simulink model "chap8_6sim"  (R2015a)
settings: Solver=ode45  StartTime=0.0  StopTime=30  RelTol=1e-3
settings Model: Creator=zhr  LastModifiedBy=zhr

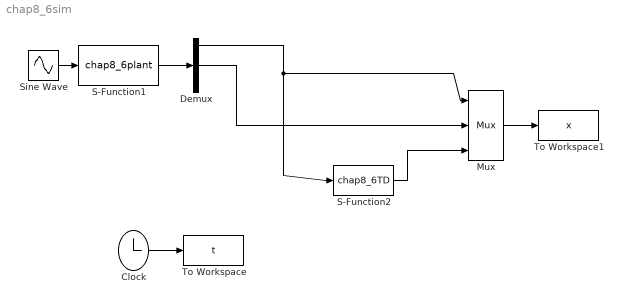
== system chap8_6sim ==
  Clock : Clock
  Demux : Demux  Outputs=3
  Mux : Mux  Inputs=3
  S-Function1 : S-Function  FunctionName=chap8_6plant
  S-Function2 : S-Function  FunctionName=chap8_6TD
  Sine Wave : Sin  Amplitude=0.1  SampleTime=0
  To Workspace : ToWorkspace  VariableName=t  SampleTime=-1
  To Workspace1 : ToWorkspace  VariableName=x  SampleTime=-1
  wires:
  S-Function1/1 -> Demux/1
  Demux/1 -> S-Function2/1, Mux/1
  Demux/2 -> Mux/2
  S-Function2/1 -> Mux/3
  Sine Wave/1 -> S-Function1/1
  Clock/1 -> To Workspace/1
  Mux/1 -> To Workspace1/1
